simulink model "PTOSwt"  (R2016b)
settings: Solver=VariableStepAuto  StartTime=0.0  StopTime=10.0  RelTol=1e-3
settings Model: Creator=jiakui  LastModifiedBy=jiakui

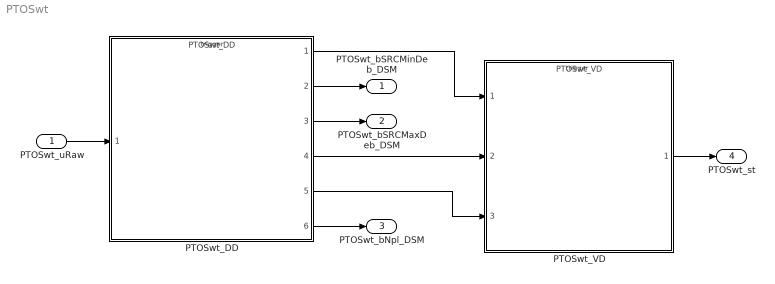
== system PTOSwt ==
  PTOSwt_uRaw : Inport  Tag=mv  Description=Raw input voltage value for PTO switch  OutMin=0  OutMax=5000  OutDataTypeStr=Ad_mv
  PTOSwt_DD : ModelReference  ModelNameDialog=PTOSwt_DD  SimulationMode=Normal  ModelReferenceVersion=1.17  TriggerPortName=function  TriggerPortTriggerType=function-call  TriggerPortStatesWhenEnabling=held
  PTOSwt_VD : ModelReference  ModelNameDialog=PTOSwt_VD  SimulationMode=Normal  ModelReferenceVersion=1.10  TriggerPortName=function  TriggerPortTriggerType=function-call  TriggerPortStatesWhenEnabling=held
  PTOSwt_bSRCMinDeb_DSM : Outport  Description="error state \"DFC_MinPTOSwt\""  OutMin=0  OutMax=1  OutDataTypeStr=boolean
  PTOSwt_bSRCMaxDeb_DSM : Outport  Description="error state \"DFC_MaxPTOSwt\""  Port=2  OutMin=0  OutMax=1  OutDataTypeStr=boolean
  PTOSwt_bNpl_DSM : Outport  Description="error state \"DFC_NplPTOSwt\""  Port=3  OutMin=0  OutMax=1  OutDataTypeStr=boolean
  PTOSwt_st : Outport  Description=Power Take-off switch current state for a specific input voltage  Port=4  OutMin=0  OutMax=255  OutDataTypeStr=State_uint8
  wires:
  PTOSwt_uRaw/1 -> PTOSwt_DD/1
  PTOSwt_DD/1 -> PTOSwt_VD/1
  PTOSwt_DD/2 -> PTOSwt_bSRCMinDeb_DSM/1
  PTOSwt_DD/3 -> PTOSwt_bSRCMaxDeb_DSM/1
  PTOSwt_DD/4 -> PTOSwt_VD/2
  PTOSwt_DD/6 -> PTOSwt_bNpl_DSM/1
  PTOSwt_DD/5 -> PTOSwt_VD/3
  PTOSwt_VD/1 -> PTOSwt_st/1
